simulink model "ContoleLateralApplication_atual"  (R2021a)
settings: Solver=ode23tb  StartTime=0.0  StopTime=TME.Simulation  FixedStep=.001  RelTol=1e-3  EnableMultiTasking=on
StartFcn:
  | %tic
StopFcn:
  | %toc
model workspace (MAT data in the model file):
  A_mu = 10
  B_reff = 8.386
  Cz = 7766.25
  DCT_Param : object (value not decoded)
  DLCXref = [0 6 7 14 33.5 34 42 50 60]
  DLCYref = [0 0 -4.5 -4 -3.75 1.5 0.5 0 0]
  D_reff = 0.25826
  Downshift_Speeds = [9.5625 12.9375 16.3125 19.6875 23.0625 26.4375 29.8125 33.1875 36.5625 39.9375 43.3125 46.6875 ... (28 elements, 4x7)]
  EngRevLim = 7000
  Pedal_Positions = [0.1 0.4 0.5 0.9]
  SUS : object (value not decoded)
  Upshift_Speeds = [12.9375 16.3125 19.6875 33 26.4375 29.8125 33.1875 52.5 39.9375 43.3125 46.6875 77.25 ... (28 elements, 4x7)]
  VEH : object (value not decoded)
  V_o = 16.7
  V_xlow = 1
  WH : object (value not decoded)
  a = 1.4
  alpha_max = 1.5
  alpha_min = -1.5
  b = 1.8
  c_zo = 209651
  epsilon = 0.1
  h = 0.134
  path : object (value not decoded)
  pio = 220000
  q_Fcx = 0
  q_Fz2 = 15.4
  q_Fzy = 0
  q_reo = 0.9974
  q_sx1 = -0.007764
  q_sx10 = 0.2824
  q_sx11 = 5.349
  q_sx12 = 0
  q_sx13 = 0
  q_sx14 = 0
  q_sx2 = 1.1915
  q_sx3 = 0.013948
  q_sx4 = 4.912
  q_sx5 = 1.02
  q_sx6 = 22.83
  q_sx7 = 0.7104
  q_sx8 = -0.023393
  q_sx9 = 0.6581
  q_sy1 = 0.00702
  q_sy2 = 0
  q_sy3 = 0.001515
  q_sy4 = 8.514e-05
  q_sy5 = 0
  q_sy6 = 0
  q_sy7 = 0.9008
  q_sy8 = -0.4089
  q_v1 = 0.0007742
  q_v2 = 0.04667
  r_Bx1 = 12.531
  r_Bx2 = 9.532
  r_Bx3 = 0
  r_By1 = 10.615
  r_By2 = 7.705
  r_By3 = 3.433e-06
  r_By4 = 0
  r_Cx1 = 1.019
  r_Cy1 = 1.0585
  r_Ex1 = -0.4487
  r_Ex2 = -0.4726
  r_Ey1 = 0.3132
  r_Ey2 = 7.63e-06
  r_Hx1 = 0.0002374
  r_Hy1 = 0.011646
  r_Hy2 = 7.63e-06
  r_Vy1 = 0.05654
  r_Vy2 = 7.63e-06
  r_Vy3 = 0
  r_Vy4 = 99.9
  r_Vy5 = 2
  r_Vy6 = 15.814
  r_o = 0.3135
  vehWidth = 2
  w = 1
values from neighbouring files (symbols this model uses):
  C1 = 1.2801    [Data_ControleLateral_atual.m]
  C2 = 23.99    [Data_ControleLateral_atual.m]
  C3 = 0.52    [Data_ControleLateral_atual.m]
symbols that are objects in the model workspace (value not decoded): VEH
undefined symbols (not defined in the file or in its folder): Disabled, EV, GND, MTR, Right, SENSOR, STEER, WHL
libraries: autolibutils x5, vehdynlibscenariocommon x5, autolibshared x5, sim3dlib x4, vehdynlibtirecommon x2, autolibmappedmotor x2, vehdynlibviscommon x2, vehdynlibsteering x1, pid_lib x1, vehdynlibdriver x1, vehdynlibsens x1, sharedtransform x1
(part 2 of 6)

== system ContoleLateralApplication_atual/Reference Generator ==
  "VehFdbk " : Inport
  3D Engine : Subsystem  Variant=on  VariantControlMode=label  LabelModeActiveChoice=0  mask(3D Engine){engine3D=Disabled, SceneDesc=Straight road, dt3D=dt3D, defaultPos=User-specified, X_o=X_o, Y_o=Y_o, Z_o=Z_o, phi_o=phi_o, theta_o=theta_o, psi_o=psi_o}
      mask prompts: engine3D "3D Engine"; SceneDesc "Scene:"; dt3D "Engine frame rate, dt3D [s]:"; X_o "Initial longitudinal position, X_o [m]:"; Y_o "Initial lateral position, Y_o [m]:"; Z_o "Initial vertical position, Z_o [m]:"; phi_o "Initial roll angle, phi_o [rad]:"; theta_o "Initial pitch angle, theta_o [rad]:"; psi_o "Initial yaw angle, psi_o [rad]:"
      mask help: This subsystem contains the interface blocks which permit the display of the vehicle in the 3D virtual environment. Enable it to view the simulation progress, disable it to inhibit the display.
      mask init:
      | switch get_param(gcb,'engine3D')
      |     case 'Disabled'
      |         set_param(gcb,'OverrideUsingVariant','0')
      |         try
      |             set_param([bdroot '/Environment/Ground Feedback'],'OverrideUsingVariant','0')
      |         catch
      |             disp('Warning: No ground feedback sensor not set')
      |         end
      |     case 'Enabled'
      |         set_param(gcb,'OverrideUsingVariant','1')
      |         try
      |             set_param([bdroot '/Environment/Ground Feedback'],'OverrideUsingVariant','1')
      |         catch
      |             disp('Warning: No ground feedback sensor not set')
      |         end
      |     otherwise
      |         set_param(gcb,'OverrideUsingVariant','0')
      | end
      settings: AttributesFormatString=|
      | %<SceneDesc>
      | %<engine3D>
      mask Help: eval('vdynblkshelp(''vdynblks3dengine'')');
      mask TypeOptions engine3D: Enabled | Disabled
      mask Callback engine3D:
      | switch get_param(gcb,'engine3D')
      |     case 'Disabled'
      |         set_param(gcb,'OverrideUsingVariant','0')
      |     case 'Enabled'
      |        set_param(gcb,'OverrideUsingVariant','1')
      |     otherwise
      |        set_param(gcb,'OverrideUsingVariant','0')
      | end
      mask TypeOptions SceneDesc:
      | 3D Engine/Simulation 3D Engine
      | 1/SceneDesc
      mask Callback SceneDesc: [~] = vdynblks3Dsceneconfig(gcb);
      mask TypeOptions defaultPos: Recommended for scene | User-specified
      mask DialogControl engineConfig Prompt: 3D Engine Settings
      mask DialogControl posSetup Prompt: Initial vehicle position
      mask DialogControl posSetupDesc Prompt: To use these initial vehicle positions, first Apply the initial values and then click Update the model workspaces with the initial values.
      mask DialogControl setModelPos Prompt: Update model workspaces with initial values
      mask DialogControl setModelPos Callback: [~] = vdynblksmdlWSconfig(gcb);
      mask Display: disp('3D Engine')
  Reference Generator : Subsystem  Variant=on  VariantControlMode=label  VariantControl=Variant1  LabelModeActiveChoice=4
  " Vis" : Outport  VectorParamsAs1DForOutWhenUnconnected=off
  " Ref" : Outport  Port=2  VectorParamsAs1DForOutWhenUnconnected=off
  " Fdbk" : Outport  Port=3  VectorParamsAs1DForOutWhenUnconnected=off
  wires:
  "VehFdbk "/1 -> 3D Engine/1(VehFdbk), Reference Generator/1("VehFdbk ")
  Reference Generator/1(" Vis") -> " Vis"/1
  Reference Generator/2(" Ref") -> " Ref"/1
  Reference Generator/3(" Fdbk") -> " Fdbk"/1

== system ContoleLateralApplication_atual/Tire2Veh ==
  Wheel : Inport
  Bus Selector7 : BusSelector  OutputSignals=omega,Fx,Re,z,zdot,Kappa,Alpha
  Dead Zone2 : DeadZone  LowerValue=-5  UpperValue=5  ZeroCross=off  SaturateOnIntegerOverflow=on
  Demux : Demux  Outputs=[2,2]
  Re : Terminator
  Unary Minus1 : UnaryMinus
  Unary Minus2 : UnaryMinus
  zdot : Terminator
  FwF : Outport  VectorParamsAs1DForOutWhenUnconnected=off
  FwR : Outport  Port=2  VectorParamsAs1DForOutWhenUnconnected=off
  z : Outport  Port=3  VectorParamsAs1DForOutWhenUnconnected=off
  omega : Outport  Port=4  VectorParamsAs1DForOutWhenUnconnected=off
  kappa : Outport  Port=5  VectorParamsAs1DForOutWhenUnconnected=off
  alpha : Outport  Port=6  VectorParamsAs1DForOutWhenUnconnected=off
  wires:
  Bus Selector7/2 -> Dead Zone2/1  "<Fx>"
  Dead Zone2/1 -> Demux/1  "Fx"
  Demux/1 -> FwF/1
  Wheel/1 -> Bus Selector7/1
  Bus Selector7/1 -> omega/1  "<omega>"
  Bus Selector7/5 -> Unary Minus2/1  "<zdot>"
  Bus Selector7/4 -> Unary Minus1/1  "<z>"
  Unary Minus1/1 -> z/1  "z"
  Demux/2 -> FwR/1
  Bus Selector7/6 -> kappa/1  "<Kappa>"
  Unary Minus2/1 -> zdot/1  "zdot"
  Bus Selector7/3 -> Re/1  "<Re>"
  Bus Selector7/7 -> alpha/1  "<Alpha>"
